simulink model "augmented_model"  (R2025a)
settings: Solver=VariableStepAuto  StartTime=0.0  StopTime=10.0  RelTol=1e-3
undefined symbols (not defined in the file or in its folder): Ar, Br, Cr, Dr
libraries: cstblocks x3
settings Model: Creator=asus  LastModifiedBy=asus
settings OptimizationCC: DefaultParameterBehavior=Inlined
settings DebuggingCC: InitInArrayFormatMsg=none

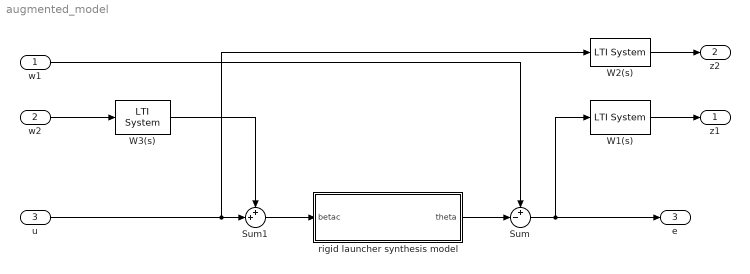
== system augmented_model ==
  w1 : Inport
  w2 : Inport  Port=2
  u : Inport  Port=3
  Sum : Sum  Inputs=+-|
  Sum1 : Sum  Inputs=++|
  W1(s) : cstblocks/LTI System  sys=sysW1  IC=[]  PadeOrder=0
  W2(s) : cstblocks/LTI System  sys=sysW2  IC=[]  PadeOrder=0
  W3(s) : cstblocks/LTI System  sys=sysW3  IC=[]  PadeOrder=0
  rigid launcher synthesis model : Subsystem
  z1 : Outport
  z2 : Outport  Port=2
  e : Outport  Port=3
  wires:
  rigid launcher synthesis model/1(theta) -> Sum/2
  Sum1/1 -> rigid launcher synthesis model/1(betac)
  u/1 -> W2(s)/1, Sum1/2
  Sum/1 -> W1(s)/1, e/1
  W1(s)/1 -> z1/1
  W2(s)/1 -> z2/1
  W3(s)/1 -> Sum1/1
  w2/1 -> W3(s)/1
  w1/1 -> Sum/1

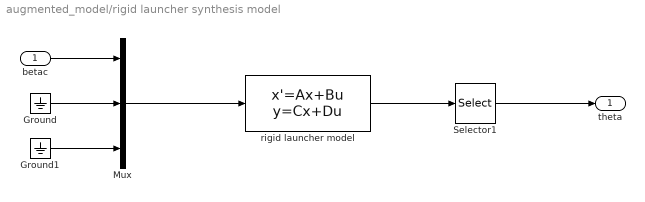
== system augmented_model/rigid launcher synthesis model ==
  betac : Inport
  Ground : Ground
  Ground1 : Ground
  Mux : Mux  Inputs=3
  Selector1 : Selector  InputPortWidth=6  IndexOptions=Index vector (dialog)  Indices=[2]  OutputSizes=1
  rigid launcher model : StateSpace  A=Ar  B=Br  C=Cr  D=Dr  InitialCondition=0
  theta : Outport
  wires:
  betac/1 -> Mux/1
  Ground1/1 -> Mux/3
  Ground/1 -> Mux/2
  Selector1/1 -> theta/1
  rigid launcher model/1 -> Selector1/1
  Mux/1 -> rigid launcher model/1
